simulink model "A_DIOL_BicopterSim"  (R2023a)
settings: Solver=ode4  StartTime=0.0  StopTime=Tend  FixedStep=Ts  RelTol=1e-3
values from neighbouring files (symbols this model uses):
  alpha_1 = 0.2    [A_DIOL_sim_runner.m]    (also in DT_A_DIOL_sim_runner.m)
  alpha_2 = 1.2    [A_DIOL_sim_runner.m]    (also in DT_A_DIOL_sim_runner.m)
  c_1 = 6    [A_DIOL_sim_runner.m]    (also in DT_A_DIOL_sim_runner.m)
  c_2 = 3    [A_DIOL_sim_runner.m]    (also in DT_A_DIOL_sim_runner.m)
  g = 9.81    [A_DIOL_sim_runner.m]    (also in DT_A_DIOL_sim_runner.m)
  gamma = 10    [A_DIOL_sim_runner.m]    (also in DT_A_DIOL_sim_runner.m)
  J = 0.05    [A_DIOL_sim_runner.m]    (also in DT_A_DIOL_sim_runner.m)
  k = place(A,B,p)    [A_DIOL_runner.m]    (also in A_DIOL_sim_runner.m; print_DE_FL.m)
  lambda = 80    [A_DIOL_sim_runner.m]    (also in DT_A_DIOL_sim_runner.m = 40)
  m = 1    [A_DIOL_sim_runner.m]    (also in DT_A_DIOL_sim_runner.m)
  Phibar_0 = ones(2,2)    [A_DIOL_sim_runner.m]    (also in DT_A_DIOL_sim_runner.m)
  Phif_0 = zeros(6,2)    [A_DIOL_sim_runner.m]    (also in DT_A_DIOL_sim_runner.m)
  Psi_int_0 = [0;0;0;0;0;0]    [A_DIOL_sim_runner.m]    (also in DT_A_DIOL_sim_runner.m)
  Theta_hat_0 = [1/m_hat_0; 1/J_hat_0]    [A_DIOL_sim_runner.m]    (also in DT_A_DIOL_sim_runner.m)
  Ts = 1e-4    (= 0.0001)    [A_DIOL_sim_runner.m]    (also in DT_A_DIOL_sim_runner.m = 0.01; trajectory_csv_generator.m)
  u1_0 = g*m_hat_0    (= 4.905)    [A_DIOL_sim_runner.m]    (also in DT_A_DIOL_sim_runner.m)
  u1_dot_0 = 0    [A_DIOL_sim_runner.m]    (also in DT_A_DIOL_sim_runner.m)
  x0 = [0.01; 0.00; 0.03; 0.02; 0.01; 0.00]    [A_DIOL_sim_runner.m]    (also in DT_A_DIOL_sim_runner.m)
  Xbar_0 = zeros(2,1)    [A_DIOL_sim_runner.m]    (also in DT_A_DIOL_sim_runner.m)
  xf_0 = x0    [A_DIOL_sim_runner.m]    (also in DT_A_DIOL_sim_runner.m)
settings Model: Creator=PhDstudent1  LastModifiedBy=Juan Augusto Paredes
settings ModelReferenceCC: EnableRefExpFcnMdlSchedulingChecks=on

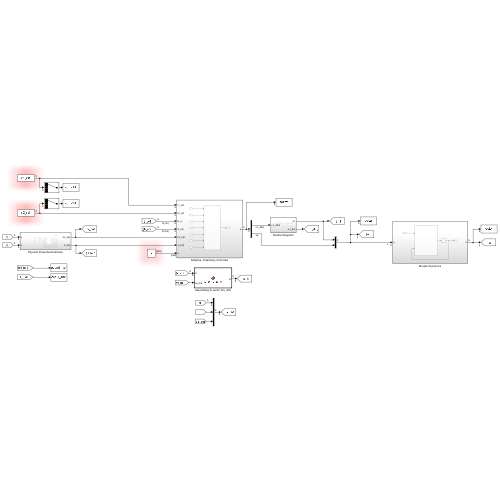
[thumbnail: Simulink's stored preview of the top-level diagram]
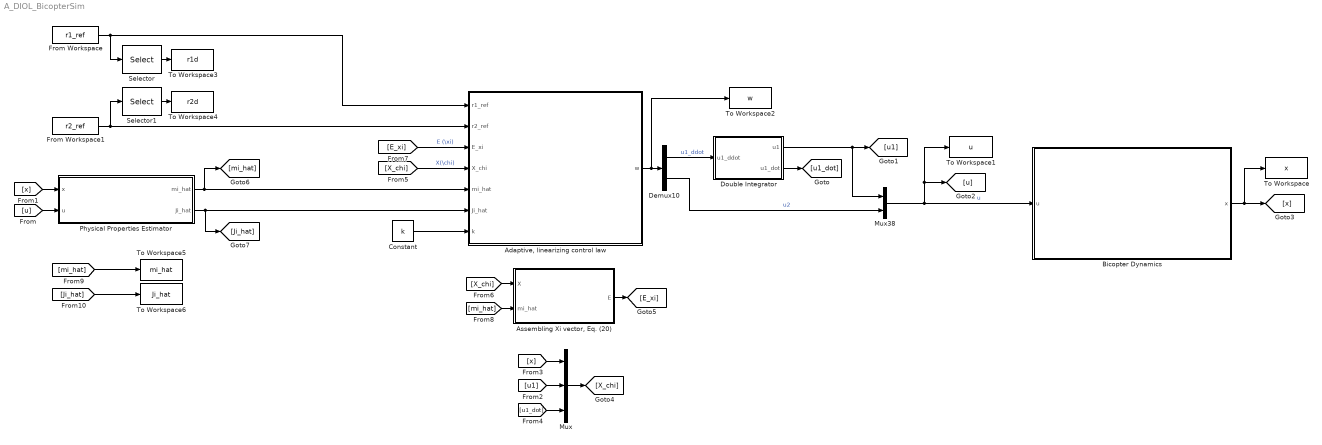
== system A_DIOL_BicopterSim ==
  "Adaptive, linearizing control law" : Subsystem
  "Assembling Xi vector, Eq. (20)" : MATLAB Function  TreatAsAtomicUnit=on
  Bicopter Dynamics : Subsystem
  Constant : Constant  Value=k
  Demux10 : Demux  Outputs=2
  Double Integrator : Subsystem
  From Workspace : FromWorkspace  VariableName=r1_ref  SampleTime=Ts
  From Workspace1 : FromWorkspace  VariableName=r2_ref  SampleTime=Ts
  Mux : Mux  Inputs=3
  Mux38 : Mux  Inputs=2
  Physical Properties Estimator : Subsystem
  Selector : Selector  InputPortWidth=5  IndexOptions=Index vector (dialog)  Indices=[1]  OutputSizes=1
  Selector1 : Selector  InputPortWidth=5  IndexOptions=Index vector (dialog)  Indices=[1]  OutputSizes=1
  To Workspace : ToWorkspace  VariableName=x  SampleTime=-1
  To Workspace1 : ToWorkspace  VariableName=u  SampleTime=-1
  To Workspace2 : ToWorkspace  VariableName=w  SampleTime=-1
  To Workspace3 : ToWorkspace  VariableName=r1d  SampleTime=-1
  To Workspace4 : ToWorkspace  VariableName=r2d  SampleTime=-1
  To Workspace5 : ToWorkspace  VariableName=mi_hat  SampleTime=-1
  To Workspace6 : ToWorkspace  VariableName=Ji_hat  SampleTime=-1
  wires:
  Mux38/1 -> Bicopter Dynamics/1(u), To Workspace1/1, [u]  "u"
  Constant/1 -> "Adaptive, linearizing control law"/7(k)
  "Adaptive, linearizing control law"/1(w) -> To Workspace2/1, Demux10/1
  [E_xi] -> "Adaptive, linearizing control law"/3(E_xi)  "E (\\xi)"
  [X_chi] -> "Adaptive, linearizing control law"/4(X_chi)  "X(\\chi)"
  Demux10/1 -> Double Integrator/1(u1_ddot)  "u1_ddot"
  Demux10/2 -> Mux38/2  "u2"
  Double Integrator/2(u1_dot) -> [u1_dot]
  Double Integrator/1(u1) -> [u1], Mux38/1
  [u] -> Physical Properties Estimator/2(u)
  Bicopter Dynamics/1(x) -> To Workspace/1, [x]
  [x] -> Physical Properties Estimator/1(x)
  [x] -> Mux/1
  [u1] -> Mux/2
  [u1_dot] -> Mux/3
  Mux/1 -> [X_chi]
  "Assembling Xi vector, Eq. (20)"/1(E) -> [E_xi]
  [X_chi] -> "Assembling Xi vector, Eq. (20)"/1(X)
  [mi_hat] -> "Assembling Xi vector, Eq. (20)"/2(mi_hat)
  From Workspace/1 -> Selector/1, "Adaptive, linearizing control law"/1(r1_ref)
  From Workspace1/1 -> Selector1/1, "Adaptive, linearizing control law"/2(r2_ref)
  Selector/1 -> To Workspace3/1
  Selector1/1 -> To Workspace4/1
  Physical Properties Estimator/2(Ji_hat) -> [Ji_hat], "Adaptive, linearizing control law"/6(Ji_hat)
  Physical Properties Estimator/1(mi_hat) -> [mi_hat], "Adaptive, linearizing control law"/5(mi_hat)
  [Ji_hat] -> To Workspace6/1
  [mi_hat] -> To Workspace5/1

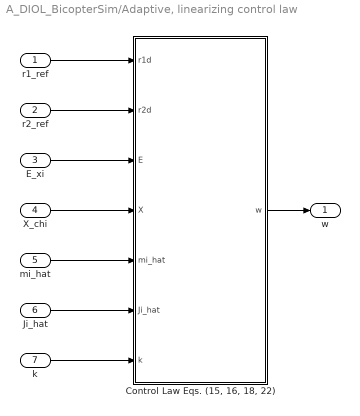
== system A_DIOL_BicopterSim/Adaptive, linearizing control law ==
  r1_ref : Inport
  r2_ref : Inport  Port=2
  E_xi : Inport  Port=3
  X_chi : Inport  Port=4
  mi_hat : Inport  Port=5
  Ji_hat : Inport  Port=6
  k : Inport  Port=7
  "Control Law Eqs. (15, 16, 18, 22)" : MATLAB Function  TreatAsAtomicUnit=on
  w : Outport
  wires:
  r1_ref/1 -> "Control Law Eqs. (15, 16, 18, 22)"/1(r1d)
  r2_ref/1 -> "Control Law Eqs. (15, 16, 18, 22)"/2(r2d)
  mi_hat/1 -> "Control Law Eqs. (15, 16, 18, 22)"/5(mi_hat)
  Ji_hat/1 -> "Control Law Eqs. (15, 16, 18, 22)"/6(Ji_hat)
  k/1 -> "Control Law Eqs. (15, 16, 18, 22)"/7(k)
  E_xi/1 -> "Control Law Eqs. (15, 16, 18, 22)"/3(E)
  X_chi/1 -> "Control Law Eqs. (15, 16, 18, 22)"/4(X)
  "Control Law Eqs. (15, 16, 18, 22)"/1(w) -> w/1

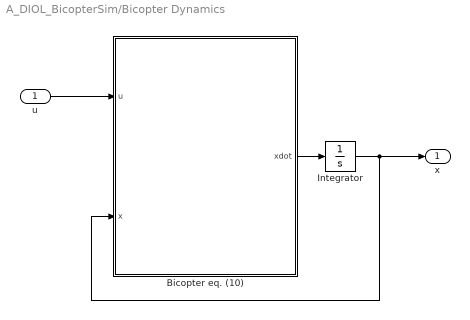
== system A_DIOL_BicopterSim/Bicopter Dynamics ==
  u : Inport
  Bicopter eq. (10) : MATLAB Function  TreatAsAtomicUnit=on
  Integrator : Integrator  InitialCondition=x0
  x : Outport
  wires:
  Bicopter eq. (10)/1(xdot) -> Integrator/1
  u/1 -> Bicopter eq. (10)/1(u)
  Integrator/1 -> x/1, Bicopter eq. (10)/2(x)

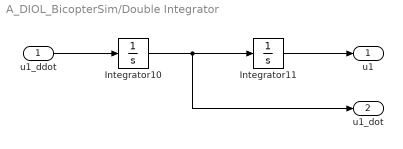
== system A_DIOL_BicopterSim/Double Integrator ==
  u1_ddot : Inport
  Integrator10 : Integrator  InitialCondition=u1_dot_0
  Integrator11 : Integrator  InitialCondition=u1_0
  u1 : Outport
  u1_dot : Outport  Port=2
  wires:
  u1_ddot/1 -> Integrator10/1
  Integrator11/1 -> u1/1
  Integrator10/1 -> u1_dot/1, Integrator11/1

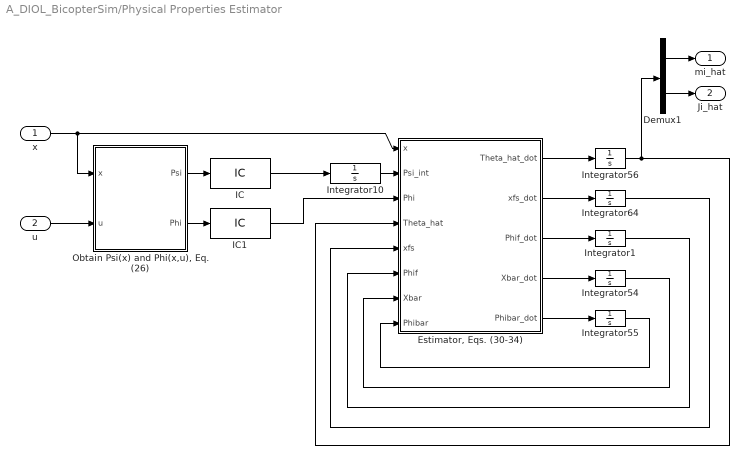
== system A_DIOL_BicopterSim/Physical Properties Estimator ==
  x : Inport
  u : Inport  Port=2
  Demux1 : Demux  Outputs=2
  "Estimator, Eqs. (30-34)" : MATLAB Function  TreatAsAtomicUnit=on
  IC : InitialCondition  Value=zeros(6,1)
  IC1 : InitialCondition  Value=zeros(6,2)
  Integrator1 : Integrator  InitialCondition=Phif_0
  Integrator10 : Integrator  InitialCondition=Psi_int_0
  Integrator54 : Integrator  InitialCondition=Xbar_0
  Integrator55 : Integrator  InitialCondition=Phibar_0
  Integrator56 : Integrator  InitialCondition=Theta_hat_0
  Integrator64 : Integrator  InitialCondition=xf_0 - x0 + Psi_int_0
  "Obtain Psi(x) and Phi(x,u), Eq. (26)" : MATLAB Function  TreatAsAtomicUnit=on
  mi_hat : Outport
  Ji_hat : Outport  Port=2
  wires:
  "Estimator, Eqs. (30-34)"/4(Xbar_dot) -> Integrator54/1
  "Estimator, Eqs. (30-34)"/5(Phibar_dot) -> Integrator55/1
  "Estimator, Eqs. (30-34)"/1(Theta_hat_dot) -> Integrator56/1
  "Estimator, Eqs. (30-34)"/2(xfs_dot) -> Integrator64/1
  "Estimator, Eqs. (30-34)"/3(Phif_dot) -> Integrator1/1
  Demux1/1 -> mi_hat/1
  Demux1/2 -> Ji_hat/1
  "Obtain Psi(x) and Phi(x,u), Eq. (26)"/1(Psi) -> IC/1
  x/1 -> "Estimator, Eqs. (30-34)"/1(x), "Obtain Psi(x) and Phi(x,u), Eq. (26)"/1(x)
  u/1 -> "Obtain Psi(x) and Phi(x,u), Eq. (26)"/2(u)
  Integrator10/1 -> "Estimator, Eqs. (30-34)"/2(Psi_int)
  Integrator56/1 -> Demux1/1, "Estimator, Eqs. (30-34)"/4(Theta_hat)
  IC/1 -> Integrator10/1
  "Obtain Psi(x) and Phi(x,u), Eq. (26)"/2(Phi) -> IC1/1
  IC1/1 -> "Estimator, Eqs. (30-34)"/3(Phi)
  Integrator55/1 -> "Estimator, Eqs. (30-34)"/8(Phibar)
  Integrator54/1 -> "Estimator, Eqs. (30-34)"/7(Xbar)
  Integrator1/1 -> "Estimator, Eqs. (30-34)"/6(Phif)
  Integrator64/1 -> "Estimator, Eqs. (30-34)"/5(xfs)

== matlab function A_DIOL_BicopterSim/Physical Properties Estimator/Obtain Psi(x) and Phi(x,u), Eq. (26) ==
  data: x input size=6; u input size=2; Psi output size=6; Phi output size=[6,2]; g parameter size=1
function [Psi, Phi] = x_2_Psi_Phi(x,u,g)
    Psi = [x(4);...
          x(5);...
          x(6);...
          0;...
          -g;...
          0];
    Phi = [0 0;...
          0 0;...
          0 0;...
          -u(1)*sin(x(3)) 0;...
          u(1)*cos(x(3)) 0;...
          0 u(2)];
end

== matlab function A_DIOL_BicopterSim/Assembling Xi vector, Eq. (20) ==
  data: X input size=8; E output size=8; mi_hat input size=1; g parameter size=1
function E = X_chi_2_E_xi(X,mi_hat,g)

m_hat = 1/mi_hat;

E = [X(1);...
    X(4);...
    -sin(X(3))*X(7)/m_hat;...
    -cos(X(3))*X(6)*X(7)/m_hat - sin(X(3))*X(8)/m_hat;...
    X(2);...
    X(5);...
    -g + cos(X(3))*X(7)/m_hat;...
    -sin(X(3))*X(6)*X(7)/m_hat + cos(X(3))*X(8)/m_hat];

== matlab function A_DIOL_BicopterSim/Adaptive, linearizing control law/Control Law Eqs. (15, 16, 18, 22) ==
  data: r1d input; r2d input; E input; X input; w output; mi_hat input; Ji_hat input; k input
function w = control_law(r1d, r2d, E, X, mi_hat, Ji_hat, k)

m_hat = 1/mi_hat;
J_hat = 1/Ji_hat;

Ed = [r1d(1:4); r2d(1:4)];
v = k*(E - Ed) + [r1d(5); r2d(5)]; % Eq. (22)

alpha_X =[-2*X(8)*cos(X(3))+X(6)*X(7)*sin(X(3)); -2*X(8)*sin(X(3))-X(6)*X(7)*cos(X(3))].*X(6)./m_hat ; % Eq. (16)
beta_X_inv = [-m_hat*sin(X(3)), m_hat*cos(X(3)); -J_hat*m_hat*cos(X(3))/X(7), -J_hat*m_hat*sin(X(3))/X(7)]; % Eq. (18)

w = beta_X_inv*(alpha_X-v); % Eq. (15)

end

== matlab function A_DIOL_BicopterSim/Bicopter Dynamics/Bicopter eq. (10) ==
  data: u input size=2; xdot output size=6; x input size=6; m parameter size=1; g parameter size=1; J parameter size=1
function xdot  = bicopter_dyn(u,x,m, g, J)

xdot = [x(4);...
        x(5);...
        x(6);...
        -sin(x(3))*u(1)/m;...
        -g+cos(x(3))*u(1)/m;...
        u(2)/J];

end

== matlab function A_DIOL_BicopterSim/Physical Properties Estimator/Estimator, Eqs. (30-34) ==
  data: Theta_hat_dot output size=2; xfs_dot output size=6; Phif_dot output size=[6,2]; x input size=6; Psi_int input size=6; Phi input size=[6, 2]; Theta_hat input size=2; xfs input size=6; Phif input size=[6,2]; Xbar input size=2; Phibar input size=[2 2]; Xbar_dot output size=2; Phibar_dot output size=[2 2]; gamma parameter size=1; lambda parameter size=1; c_1 parameter size=1; c_2 parameter size=1; alpha_1 parameter size=1; alpha_2 parameter size=1
function [Theta_hat_dot,xfs_dot,Phif_dot,...
    Xbar_dot,Phibar_dot] = estimator(x, Psi_int,Phi,...
                                        Theta_hat,xfs,Phif,Xbar,Phibar,...
                                        gamma, lambda, c_1, c_2, alpha_1, alpha_2)

%xf and Phif dynamics, Eq. (30)

xf = xfs + x - Psi_int; % xfs is an intermediate variable for calculating xf
xfs_dot=-gamma*xf;

Phif_dot=-gamma*Phif+Phi;

%Finite time estimator

Xbar_dot = Phif'*xf - lambda*Xbar; % Eq. (33)
Phibar_dot = Phif'*Phif - lambda*Phibar; % Eq. (34)
grad= Phibar*Theta_hat-Xbar; % Eq. (32)
Theta_hat_dot = -c_1*grad/(norm(grad)^(1-alpha_1))-c_2*grad/(norm(grad)^(1-alpha_2));  % Eq. (31)

end
